simulink model "foc_basic_SVPWM"  (R2025b)
settings: Solver=ode4  StartTime=0.0  StopTime=5  FixedStep=1e-5  RelTol=1e-3
libraries: slpidlib x3
settings Model: Creator=86156  LastModifiedBy=86156

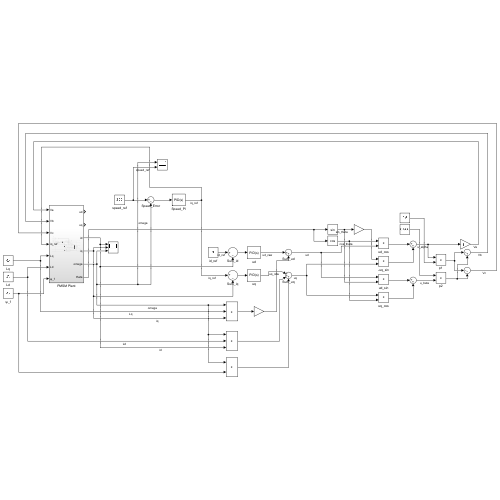
[thumbnail: Simulink's stored preview of the top-level diagram]
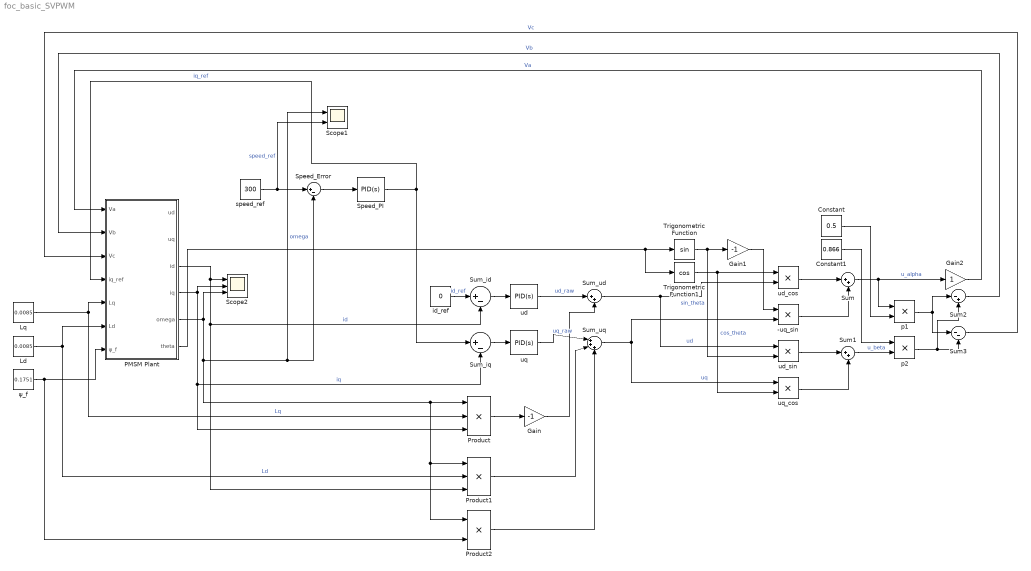
== system foc_basic_SVPWM ==
  -uq_sin : Product
  Constant : Constant  Value=0.5
  Constant1 : Constant  Value=0.866
  Gain : Gain  Gain=-1
  Gain1 : Gain  Gain=-1
  Gain2 : Gain
  Ld : Constant  Value=0.0085
  Lq : Constant  Value=0.0085
  PMSM Plant : Subsystem
  Product : Product  Inputs=3
  Product1 : Product  Inputs=3
  Product2 : Product
  Scope1 : Scope  NumInputPorts=2
      settings: ActiveDisplayYMinimum=-19.724436766679965  ActiveDisplayYMaximum=446.22820788137739
  Scope2 : Scope  NumInputPorts=3
      settings: ActiveDisplayYMinimum=-314.47884246711953  ActiveDisplayYMaximum=240.84611189264956  DataLoggingVariableName=ScopeData2
  Speed_Error : Sum  Inputs=|+-
  Speed_PI : slpidlib/PID Controller  Controller=PID  Form=Parallel  TimeDomain=Continuous-time  UseExternalTs=off  SampleTime=-1  IntegratorMethod=Forward Euler  FilterMethod=Forward Euler  ControllerParametersSource=internal  P=0.3  I=8  UseKiTs=off  D=0  UseExternalDerivativeSource=off  N=100  UseFilter=on  TunerSelectOption=Transfer Function Based (PID Tuner App)  InitialConditionSource=internal  InitialConditionForIntegrator=0  InitialConditionForFilter=0  DifferentiatorICPrevScaledInput=0  ExternalReset=none  TrackingMode=off  Kt=1  LimitOutput=off  SatLimitsSource=internal  UpperSaturationLimit=inf  LowerSaturationLimit=-inf  LinearizeAsGain=on  AntiWindupMode=none  Kb=1  LimitIntegrator=off  UpperIntegratorSaturationLimit=inf  LowerIntegratorSaturationLimit=-inf  POutMin=[]  POutMax=[]  IOutMin=[]  IOutMax=[]  DOutMin=[]  DOutMax=[]  NOutMin=[]  NOutMax=[]  SumOutMin=[]  SumOutMax=[]  SaturationOutMin=[]  SaturationOutMax=[]  PParamMin=[]  PParamMax=[]  IParamMin=[]  IParamMax=[]  DParamMin=[]  DParamMax=[]  NParamMin=[]  NParamMax=[]  KbParamMin=[]  KbParamMax=[]  KtParamMin=[]  KtParamMax=[]  KbOutMin=[]  KbOutMax=[]  KtOutMin=[]  KtOutMax=[]  IntegratorOutMin=[]  IntegratorOutMax=[]  FilterOutMin=[]  FilterOutMax=[]  SumI1OutMin=[]  SumI1OutMax=[]  SumI2OutMin=[]  SumI2OutMax=[]  SumI3OutMin=[]  SumI3OutMax=[]  SumI4OutMin=[]  SumI4OutMax=[]  SumDOutMin=[]  SumDOutMax=[]  DifferentiatorOutMin=[]  DifferentiatorOutMax=[]  FilterDiffOutCoefMin=[]  FilterDiffOutCoefMax=[]  ReciprocalOutMin=[]  ReciprocalOutMax=[]  SumDenOutMin=[]  SumDenOutMax=[]  SumNumOutMin=[]  SumNumOutMax=[]  DivideOutMin=[]  DivideOutMax=[]  UdiffTsProdOutMin=[]  UdiffTsProdOutMax=[]  NTsProdOutMin=[]  NTsProdOutMax=[]  UintegralTsProdOutMin=[]  UintegralTsProdOutMax=[]  UngainTsProdOutMin=[]  UngainTsProdOutMax=[]  ClampingZeroOutDataTypeStr=Inherit: Inherit via back propagation  ClampingZeroOutMin=[]  ClampingZeroOutMax=[]  FilterDenConstantOutDataTypeStr=Inherit: Inherit via back propagation  FilterDenConstantOutMin=[]  FilterDenConstantOutMax=[]  PCopyOutDataTypeStr=Inherit: Inherit via back propagation  PCopyOutMin=[]  PCopyOutMax=[]  NCopyOutDataTypeStr=Inherit: Inherit via back propagation  NCopyOutMin=[]  NCopyOutMax=[]  IntegratorContinuousStateAttributes=''  IntegratorStateMustResolveToSignalObject=off  IntegratorRTWStateStorageClass=Auto  FilterContinuousStateAttributes=''  FilterStateMustResolveToSignalObject=off  FilterRTWStateStorageClass=Auto  ParallelPVariant=InternalParameters  IdealPVariant=Disabled  IVariant=InternalParameters  DVariant=InternalParameters  IntegratorVariant=Continuous  SatVariant=Disabled  AWVariant=Passthrough  PCopyVariant=Disabled  TRVariant=Disabled  FdbkBlocksVariant=Forward  IdealPFdbkVariant=Disabled  SatFdbkVariant=Disabled  DerivativeFilterVariant=ContFilter  NVariant=InternalParameters  NCopyVariant=Disabled  FilterICVariant=InternalICsFilter  IntegratorICVariant=InternalICs  ExternalResetVariant=Disabled  TRSumVariant=Passthrough  SumFdbkVariant=Disabled  SumVariant=Sum_PID  TsampFilterVariant=InternalTs  TsampNgainVariant=Passthrough  TsampIntegralVariant=Disabled_SignalSpec  ExternalSaturationOutDataTypeStr=Inherit: Same as second input  DerivativeSourceVariant=ErrorSignal  PreIntVariant=InternalPreInt
  Sum : Sum  Inputs=|++
  Sum1 : Sum  Inputs=|++
  Sum2 : Sum  Inputs=|-+
  Sum3 : Sum  Inputs=|--
  Sum_id : Sum  Inputs=|+-
  Sum_iq : Sum  Inputs=|+-
  Sum_ud : Sum  Inputs=|++
  Sum_uq : Sum  Inputs=|+++
  Trigonometric Function : Trigonometry
  Trigonometric Function1 : Trigonometry  Operator=cos
  id_ref : Constant  Value=0
  p1 : Product
  p2 : Product
  speed_ref : Constant  Value=300
  ud : slpidlib/PID Controller  Controller=PID  Form=Parallel  TimeDomain=Continuous-time  UseExternalTs=off  SampleTime=-1  IntegratorMethod=Forward Euler  FilterMethod=Forward Euler  ControllerParametersSource=internal  P=10  I=200  UseKiTs=off  D=0  UseExternalDerivativeSource=off  N=100  UseFilter=on  TunerSelectOption=Transfer Function Based (PID Tuner App)  InitialConditionSource=internal  InitialConditionForIntegrator=0  InitialConditionForFilter=0  DifferentiatorICPrevScaledInput=0  ExternalReset=none  TrackingMode=off  Kt=1  LimitOutput=off  SatLimitsSource=internal  UpperSaturationLimit=inf  LowerSaturationLimit=-inf  LinearizeAsGain=on  AntiWindupMode=none  Kb=1  LimitIntegrator=off  UpperIntegratorSaturationLimit=inf  LowerIntegratorSaturationLimit=-inf  POutMin=[]  POutMax=[]  IOutMin=[]  IOutMax=[]  DOutMin=[]  DOutMax=[]  NOutMin=[]  NOutMax=[]  SumOutMin=[]  SumOutMax=[]  SaturationOutMin=[]  SaturationOutMax=[]  PParamMin=[]  PParamMax=[]  IParamMin=[]  IParamMax=[]  DParamMin=[]  DParamMax=[]  NParamMin=[]  NParamMax=[]  KbParamMin=[]  KbParamMax=[]  KtParamMin=[]  KtParamMax=[]  KbOutMin=[]  KbOutMax=[]  KtOutMin=[]  KtOutMax=[]  IntegratorOutMin=[]  IntegratorOutMax=[]  FilterOutMin=[]  FilterOutMax=[]  SumI1OutMin=[]  SumI1OutMax=[]  SumI2OutMin=[]  SumI2OutMax=[]  SumI3OutMin=[]  SumI3OutMax=[]  SumI4OutMin=[]  SumI4OutMax=[]  SumDOutMin=[]  SumDOutMax=[]  DifferentiatorOutMin=[]  DifferentiatorOutMax=[]  FilterDiffOutCoefMin=[]  FilterDiffOutCoefMax=[]  ReciprocalOutMin=[]  ReciprocalOutMax=[]  SumDenOutMin=[]  SumDenOutMax=[]  SumNumOutMin=[]  SumNumOutMax=[]  DivideOutMin=[]  DivideOutMax=[]  UdiffTsProdOutMin=[]  UdiffTsProdOutMax=[]  NTsProdOutMin=[]  NTsProdOutMax=[]  UintegralTsProdOutMin=[]  UintegralTsProdOutMax=[]  UngainTsProdOutMin=[]  UngainTsProdOutMax=[]  ClampingZeroOutDataTypeStr=Inherit: Inherit via back propagation  ClampingZeroOutMin=[]  ClampingZeroOutMax=[]  FilterDenConstantOutDataTypeStr=Inherit: Inherit via back propagation  FilterDenConstantOutMin=[]  FilterDenConstantOutMax=[]  PCopyOutDataTypeStr=Inherit: Inherit via back propagation  PCopyOutMin=[]  PCopyOutMax=[]  NCopyOutDataTypeStr=Inherit: Inherit via back propagation  NCopyOutMin=[]  NCopyOutMax=[]  IntegratorContinuousStateAttributes=''  IntegratorStateMustResolveToSignalObject=off  IntegratorRTWStateStorageClass=Auto  FilterContinuousStateAttributes=''  FilterStateMustResolveToSignalObject=off  FilterRTWStateStorageClass=Auto  ParallelPVariant=InternalParameters  IdealPVariant=Disabled  IVariant=InternalParameters  DVariant=InternalParameters  IntegratorVariant=Continuous  SatVariant=Disabled  AWVariant=Passthrough  PCopyVariant=Disabled  TRVariant=Disabled  FdbkBlocksVariant=Forward  IdealPFdbkVariant=Disabled  SatFdbkVariant=Disabled  DerivativeFilterVariant=ContFilter  NVariant=InternalParameters  NCopyVariant=Disabled  FilterICVariant=InternalICsFilter  IntegratorICVariant=InternalICs  ExternalResetVariant=Disabled  TRSumVariant=Passthrough  SumFdbkVariant=Disabled  SumVariant=Sum_PID  TsampFilterVariant=InternalTs  TsampNgainVariant=Passthrough  TsampIntegralVariant=Disabled_SignalSpec  ExternalSaturationOutDataTypeStr=Inherit: Same as second input  DerivativeSourceVariant=ErrorSignal  PreIntVariant=InternalPreInt
  ud_cos : Product
  ud_sin : Product
  uq : slpidlib/PID Controller  Controller=PID  Form=Parallel  TimeDomain=Continuous-time  UseExternalTs=off  SampleTime=-1  IntegratorMethod=Forward Euler  FilterMethod=Forward Euler  ControllerParametersSource=internal  P=10  I=200  UseKiTs=off  D=0  UseExternalDerivativeSource=off  N=100  UseFilter=on  TunerSelectOption=Transfer Function Based (PID Tuner App)  InitialConditionSource=internal  InitialConditionForIntegrator=0  InitialConditionForFilter=0  DifferentiatorICPrevScaledInput=0  ExternalReset=none  TrackingMode=off  Kt=1  LimitOutput=off  SatLimitsSource=internal  UpperSaturationLimit=inf  LowerSaturationLimit=-inf  LinearizeAsGain=on  AntiWindupMode=none  Kb=1  LimitIntegrator=off  UpperIntegratorSaturationLimit=inf  LowerIntegratorSaturationLimit=-inf  POutMin=[]  POutMax=[]  IOutMin=[]  IOutMax=[]  DOutMin=[]  DOutMax=[]  NOutMin=[]  NOutMax=[]  SumOutMin=[]  SumOutMax=[]  SaturationOutMin=[]  SaturationOutMax=[]  PParamMin=[]  PParamMax=[]  IParamMin=[]  IParamMax=[]  DParamMin=[]  DParamMax=[]  NParamMin=[]  NParamMax=[]  KbParamMin=[]  KbParamMax=[]  KtParamMin=[]  KtParamMax=[]  KbOutMin=[]  KbOutMax=[]  KtOutMin=[]  KtOutMax=[]  IntegratorOutMin=[]  IntegratorOutMax=[]  FilterOutMin=[]  FilterOutMax=[]  SumI1OutMin=[]  SumI1OutMax=[]  SumI2OutMin=[]  SumI2OutMax=[]  SumI3OutMin=[]  SumI3OutMax=[]  SumI4OutMin=[]  SumI4OutMax=[]  SumDOutMin=[]  SumDOutMax=[]  DifferentiatorOutMin=[]  DifferentiatorOutMax=[]  FilterDiffOutCoefMin=[]  FilterDiffOutCoefMax=[]  ReciprocalOutMin=[]  ReciprocalOutMax=[]  SumDenOutMin=[]  SumDenOutMax=[]  SumNumOutMin=[]  SumNumOutMax=[]  DivideOutMin=[]  DivideOutMax=[]  UdiffTsProdOutMin=[]  UdiffTsProdOutMax=[]  NTsProdOutMin=[]  NTsProdOutMax=[]  UintegralTsProdOutMin=[]  UintegralTsProdOutMax=[]  UngainTsProdOutMin=[]  UngainTsProdOutMax=[]  ClampingZeroOutDataTypeStr=Inherit: Inherit via back propagation  ClampingZeroOutMin=[]  ClampingZeroOutMax=[]  FilterDenConstantOutDataTypeStr=Inherit: Inherit via back propagation  FilterDenConstantOutMin=[]  FilterDenConstantOutMax=[]  PCopyOutDataTypeStr=Inherit: Inherit via back propagation  PCopyOutMin=[]  PCopyOutMax=[]  NCopyOutDataTypeStr=Inherit: Inherit via back propagation  NCopyOutMin=[]  NCopyOutMax=[]  IntegratorContinuousStateAttributes=''  IntegratorStateMustResolveToSignalObject=off  IntegratorRTWStateStorageClass=Auto  FilterContinuousStateAttributes=''  FilterStateMustResolveToSignalObject=off  FilterRTWStateStorageClass=Auto  ParallelPVariant=InternalParameters  IdealPVariant=Disabled  IVariant=InternalParameters  DVariant=InternalParameters  IntegratorVariant=Continuous  SatVariant=Disabled  AWVariant=Passthrough  PCopyVariant=Disabled  TRVariant=Disabled  FdbkBlocksVariant=Forward  IdealPFdbkVariant=Disabled  SatFdbkVariant=Disabled  DerivativeFilterVariant=ContFilter  NVariant=InternalParameters  NCopyVariant=Disabled  FilterICVariant=InternalICsFilter  IntegratorICVariant=InternalICs  ExternalResetVariant=Disabled  TRSumVariant=Passthrough  SumFdbkVariant=Disabled  SumVariant=Sum_PID  TsampFilterVariant=InternalTs  TsampNgainVariant=Passthrough  TsampIntegralVariant=Disabled_SignalSpec  ExternalSaturationOutDataTypeStr=Inherit: Same as second input  DerivativeSourceVariant=ErrorSignal  PreIntVariant=InternalPreInt
  uq_cos : Product
  ψ_f : Constant  Value=0.1751
  wires:
  PMSM Plant/3(id) -> Sum_id/2, Product1/3, Scope2/1  "id"
  PMSM Plant/4(iq) -> Product/3, Sum_iq/2, Scope2/2  "iq"
  PMSM Plant/5(omega) -> Scope2/3, Product2/1, Product1/1, Product/1, Scope1/1, Speed_Error/2  "omega"
  speed_ref/1 -> Scope1/2, Speed_Error/1  "speed_ref"
  Speed_Error/1 -> Speed_PI/1
  Speed_PI/1 -> Sum_iq/1, PMSM Plant/4(iq_ref)  "iq_ref"
  id_ref/1 -> Sum_id/1  "id_ref"
  Sum_id/1 -> ud/1
  Sum_iq/1 -> uq/1
  ud/1 -> Sum_ud/1  "ud_raw"
  uq/1 -> Sum_uq/1  "uq_raw"
  Lq/1 -> Product/2, PMSM Plant/5(Lq)  "Lq"
  Ld/1 -> Product1/2, PMSM Plant/6(Ld)  "Ld"
  Product/1 -> Gain/1
  ψ_f/1 -> Product2/2, PMSM Plant/7(ψ_f)
  Gain/1 -> Sum_ud/2
  Product1/1 -> Sum_uq/2
  Product2/1 -> Sum_uq/3
  Sum_ud/1 -> ud_sin/1, ud_cos/2  "ud"
  Sum_uq/1 -> uq_cos/1, -uq_sin/2  "uq"
  PMSM Plant/6(theta) -> Trigonometric Function1/1, Trigonometric Function/1
  Trigonometric Function/1 -> ud_sin/2, Gain1/1  "sin_theta"
  Trigonometric Function1/1 -> uq_cos/2, ud_cos/1  "cos_theta"
  Gain1/1 -> -uq_sin/1
  ud_cos/1 -> Sum/1
  -uq_sin/1 -> Sum/2
  ud_sin/1 -> Sum1/1
  uq_cos/1 -> Sum1/2
  Sum/1 -> Gain2/1, p1/1  "u_alpha"
  Sum1/1 -> p2/2  "u_beta"
  Constant/1 -> p1/2
  Constant1/1 -> p2/1
  p1/1 -> Sum2/1, Sum3/1
  p2/1 -> Sum3/2, Sum2/2
  Sum2/1 -> PMSM Plant/2(Vb)  "Vb"
  Sum3/1 -> PMSM Plant/3(Vc)  "Vc"
  Gain2/1 -> PMSM Plant/1(Va)  "Va"

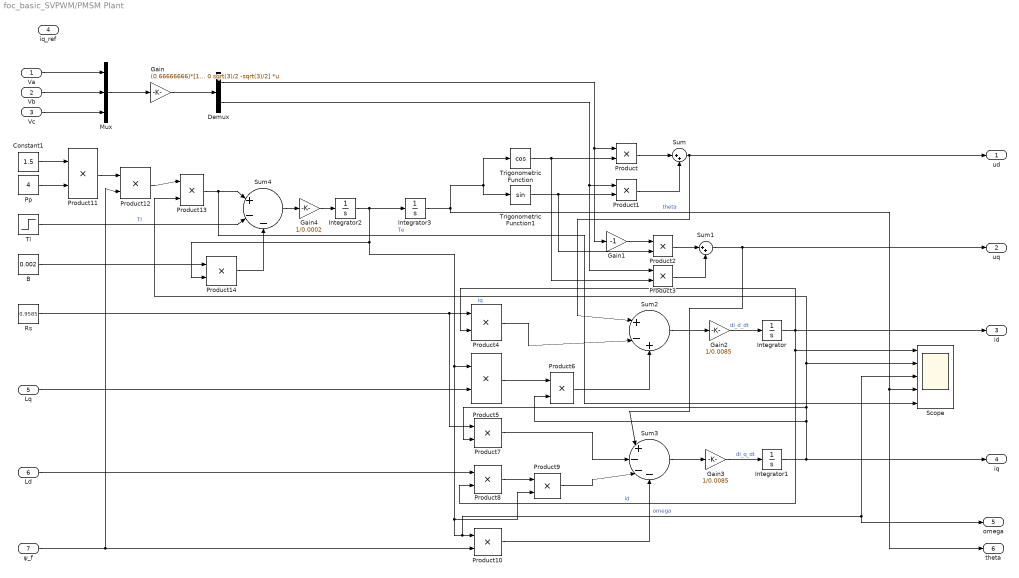
== system foc_basic_SVPWM/PMSM Plant ==
  Va : Inport
  Vb : Inport  Port=2
  Vc : Inport  Port=3
  iq_ref : Inport  Port=4
  Lq : Inport  Port=5
  Ld : Inport  Port=6
  ψ_f : Inport  Port=7
  B : Constant  Value=0.002
  Constant1 : Constant  Value=1.5
  Demux : Demux  Outputs=2
  Gain : Gain  Gain=(0.66666666)*[1 -0.5 -0.5; 0 sqrt(3)/2 -sqrt(3)/2]  Multiplication=Matrix(K*u)
  Gain1 : Gain  Gain=-1
  Gain2 : Gain  Gain=1/0.0085
  Gain3 : Gain  Gain=1/0.0085
  Gain4 : Gain  Gain=1/0.0002
  Integrator{,1..3} (4 alike) : Integrator
  Mux : Mux  Inputs=3
  Pp : Constant  Value=4
  Product{,1..14} (15 alike) : Product
  Rs : Constant  Value=0.9585
  Scope : Scope  NumInputPorts=5
      settings: ActiveDisplayYMinimum=-2.1670104752635118E+6  ActiveDisplayYMaximum=2.1159253160519088E+6  DataLoggingVariableName=ScopeData3
  Sum : Sum  Inputs=|++
  Sum1 : Sum  Inputs=|++
  Sum2 : Sum  Inputs=|+-+
  Sum3 : Sum  Inputs=|+---
  Sum4 : Sum  Inputs=|+--
  Tl : Step  After=5  SampleTime=0
  Trigonometric Function : Trigonometry  Operator=cos
  Trigonometric Function1 : Trigonometry
  ud : Outport
  uq : Outport  Port=2
  id : Outport  Port=3
  iq : Outport  Port=4
  omega : Outport  Port=5
  theta : Outport  Port=6
  wires:
  Va/1 -> Mux/1
  Vb/1 -> Mux/2
  Vc/1 -> Mux/3
  Mux/1 -> Gain/1
  Gain/1 -> Demux/1
  Demux/1 -> Gain1/1, Product/1
  Demux/2 -> Product3/1, Product1/1
  Trigonometric Function1/1 -> Product2/2, Product1/2
  Trigonometric Function/1 -> Product3/2, Product/2
  Product/1 -> Sum/1
  Product1/1 -> Sum/2
  Sum/1 -> ud/1, Sum2/1
  Gain1/1 -> Product2/1
  Product2/1 -> Sum1/1
  Product3/1 -> Sum1/2
  Sum1/1 -> Sum3/1, uq/1
  Rs/1 -> Product7/1, Product4/1
  Lq/1 -> Product5/2
  Product5/1 -> Product6/1
  Product4/1 -> Sum2/2
  Product6/1 -> Sum2/3
  Sum2/1 -> Gain2/1
  Ld/1 -> Product8/1
  Product7/1 -> Sum3/2
  Product8/1 -> Product9/1
  Product9/1 -> Sum3/3
  Product10/1 -> Sum3/4
  Sum3/1 -> Gain3/1
  Gain2/1 -> Integrator/1  "di_d_dt"
  Gain3/1 -> Integrator1/1  "di_q_dt"
  Integrator/1 -> Product8/2, Scope/1, Product4/2, id/1  "id"
  Integrator1/1 -> Product13/2, Scope/2, Product7/2, Product6/2, iq/1  "iq"
  Integrator3/1 -> Trigonometric Function/1, Trigonometric Function1/1, Scope/4, theta/1  "theta"
  Constant1/1 -> Product11/1
  Product11/1 -> Product12/1
  ψ_f/1 -> Product10/2, Product12/2
  Product12/1 -> Product13/1
  Product13/1 -> Sum4/1, Scope/5  "Te"
  Tl/1 -> Sum4/2  "Tl"
  B/1 -> Product14/1
  Integrator2/1 -> Product10/1, Scope/3, omega/1, Product9/2, Product5/1, Product14/2, Integrator3/1  "omega"
  Product14/1 -> Sum4/3
  Sum4/1 -> Gain4/1
  Gain4/1 -> Integrator2/1
  Pp/1 -> Product11/2
